simulink model "mode_adaptive(incomplete)"  (R2022a)
settings: Solver=VariableStepAuto  StartTime=0.0  StopTime=10.0  RelTol=1e-3
libraries: frdmk64flib x1
settings Model: Creator=aldra  LastModifiedBy=aldra

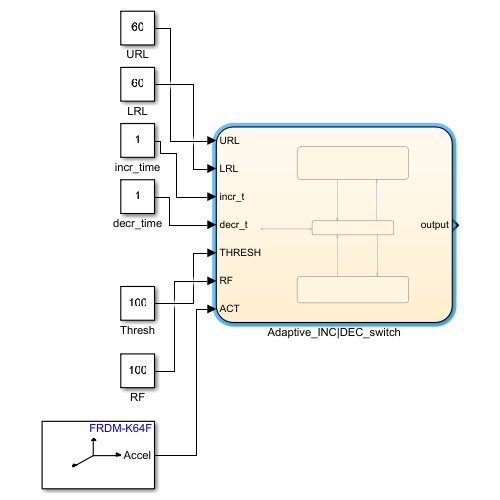
[thumbnail: Simulink's stored preview of the top-level diagram]
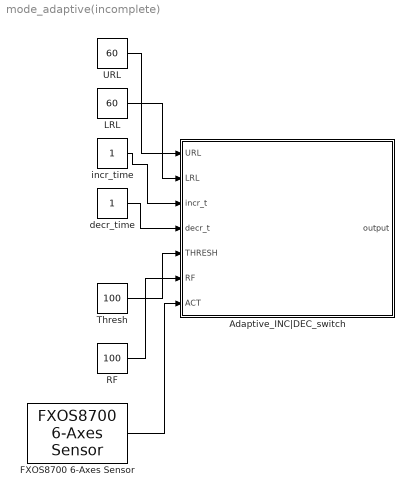
== system mode_adaptive(incomplete) ==
  Adaptive_INC|DEC_switch : Stateflow chart  TreatAsAtomicUnit=on
  FXOS8700 6-Axes Sensor : frdmk64flib/FXOS8700 6-Axes Sensor  Activesensor=Accelerometer only  ODR=800Hz  HybridODR=400Hz  Accelfullrange=-4g to +4g  SampleTime=-1
  LRL : Constant  Value=60
  RF : Constant  Value=100
  Thresh : Constant  Value=100
  URL : Constant  Value=60
  decr_time : Constant
  incr_time : Constant
  wires:
  FXOS8700 6-Axes Sensor/1 -> Adaptive_INC|DEC_switch/7(ACT)
  URL/1 -> Adaptive_INC|DEC_switch/1(URL)
  LRL/1 -> Adaptive_INC|DEC_switch/2(LRL)
  incr_time/1 -> Adaptive_INC|DEC_switch/3(incr_t)
  Thresh/1 -> Adaptive_INC|DEC_switch/5(THRESH)
  RF/1 -> Adaptive_INC|DEC_switch/6(RF)
  decr_time/1 -> Adaptive_INC|DEC_switch/4(decr_t)

== stateflow chart mode_adaptive(incomplete)/Adaptive_INC|DEC_switch ==
  state ADAP_INCR_TRIGGER
    entry:
    HR_GOAL= ( LRL + (URL - LRL) / (RF*10) * ACT );
    output = ( LRL + (HR_GOAL - LRL) / (incr_t*10) );
  state STANDBY
    entry:
    HR_GOAL= ( LRL + (URL - LRL) / (RF*10) * ACT );
    CURR_HR = output
  state ADAP_DECR_TRIGGER
    entry:
    output = ( CURR_HR - (CURR_HR - LRL) / (decr_t*10) );
  ADAP_INCR_TRIGGER -> STANDBY : [ACT <= THRESH]
  STANDBY -> ADAP_INCR_TRIGGER [order 1] : [ACT > THRESH]
  (default) -> STANDBY
  ADAP_DECR_TRIGGER -> STANDBY : [ACT > THRESH]
  STANDBY -> ADAP_DECR_TRIGGER [order 2] : [ACT <= THRESH]
  data: URL input; LRL input; incr_t input; decr_t input; THRESH input; RF input; ACT input; output output
